simulink model "model"  (R2018b)
settings: Solver=VariableStepAuto  StartTime=0.0  StopTime=10.0  RelTol=1e-3
values from neighbouring files (symbols this model uses):
  dt = 0    [runScript.m]
  Vx = 0    [runScript.m]
  Vx_prev = 0    [runScript.m]
  Vy = 0    [runScript.m]
  Vy_prev = 0    [runScript.m]
  Vz = 0    [runScript.m]
  Vz_prev = 0    [runScript.m]
settings Model: Creator=Leshi  LastModifiedBy=Leshi

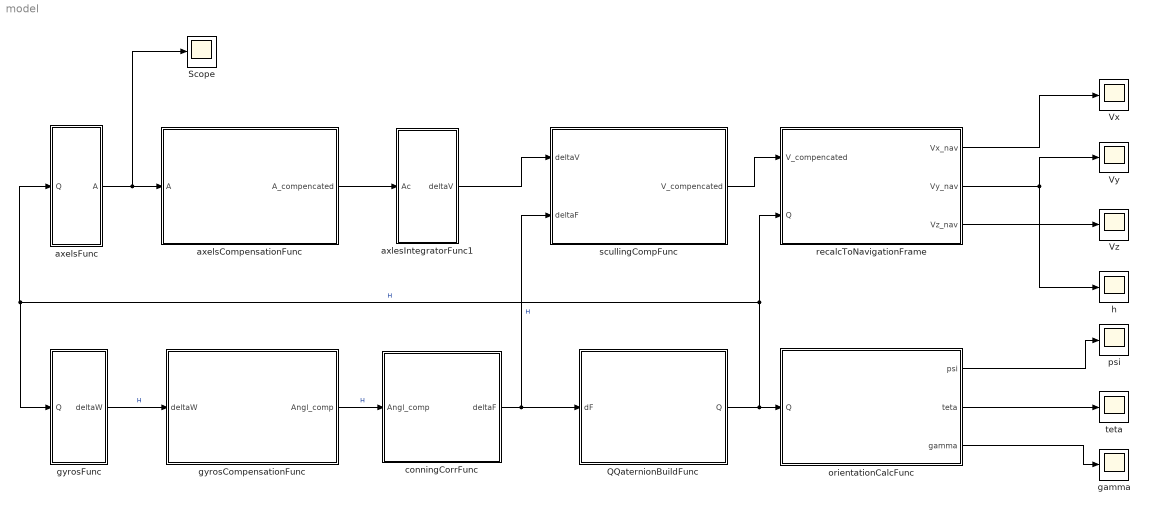
== system model ==
  QQaternionBuildFunc : MATLAB Function  TreatAsAtomicUnit=on
  Scope : Scope
  Vx : Scope
  Vy : Scope
  Vz : Scope
  axelsCompensationFunc : MATLAB Function  TreatAsAtomicUnit=on
  axelsFunc : MATLAB Function  TreatAsAtomicUnit=on
  axlesIntegratorFunc1 : MATLAB Function  TreatAsAtomicUnit=on
  conningCorrFunc : MATLAB Function  TreatAsAtomicUnit=on
  gamma : Scope
  gyrosCompensationFunc : MATLAB Function  TreatAsAtomicUnit=on
  gyrosFunc : MATLAB Function  TreatAsAtomicUnit=on
  h : Scope
  orientationCalcFunc : MATLAB Function  TreatAsAtomicUnit=on
  psi : Scope
  recalcToNavigationFrame : MATLAB Function  TreatAsAtomicUnit=on
  scullingCompFunc : MATLAB Function  TreatAsAtomicUnit=on
  teta : Scope
  wires:
  gyrosFunc/1(deltaW) -> gyrosCompensationFunc/1(deltaW)  "н"
  QQaternionBuildFunc/1(Q) -> orientationCalcFunc/1(Q), recalcToNavigationFrame/2(Q), gyrosFunc/1(Q), axelsFunc/1(Q)  "н"
  recalcToNavigationFrame/1(Vx_nav) -> Vx/1
  recalcToNavigationFrame/3(Vz_nav) -> Vz/1
  recalcToNavigationFrame/2(Vy_nav) -> h/1, Vy/1
  orientationCalcFunc/1(psi) -> psi/1
  orientationCalcFunc/2(teta) -> teta/1
  orientationCalcFunc/3(gamma) -> gamma/1
  gyrosCompensationFunc/1(Angl_comp) -> conningCorrFunc/1(Angl_comp)  "н"
  axlesIntegratorFunc1/1(deltaV) -> scullingCompFunc/1(deltaV)
  axelsFunc/1(A) -> Scope/1, axelsCompensationFunc/1(A)
  axelsCompensationFunc/1(A_compencated) -> axlesIntegratorFunc1/1(Ac)
  scullingCompFunc/1(V_compencated) -> recalcToNavigationFrame/1(V_compencated)
  conningCorrFunc/1(deltaF) -> scullingCompFunc/2(deltaF), QQaternionBuildFunc/1(dF)  "н"

== matlab function model/gyrosFunc ==
  data: deltaW output size=[1, 3]; Q input size=[1, 4]
% Give increment of anular vels
function deltaW = Gyros(Q)



Wx = awgn(0,10,'measured');
Wy = awgn(0,10,'measured');
Wz = awgn(0,10,'measured');

deltaW = [Wx, Wy, Wz];

== matlab function model/axelsFunc ==
  data: Q input size=[1, 4]; A output size=[1, 3]; g parameter
% Give pure aceleration
function A = Axels(Q, g)

[q0, q1, q2, q3] = parts(Q)
Q_ = quaternion(q0, -q1, -q2, -q3);
gCurrnet = Q * g * Q_;

Ax = awgn(gCurrnet(1),10,'measured');
Ay = awgn(gCurrnet(2),10,'measured');
Az = awgn(gCurrnet(3),10,'measured');

A = [Ax, Ay, Az];

== matlab function model/axelsCompensationFunc ==
  data: A input size=[1, 3]; A_compencated output; g parameter
function A_compencated  = AxelsCompensation(A, g)
Ax_compencated = A(1);
Ay_compencated = A(2) - g;
Az_compencated = A(3);

A_compencated = [Ax_compencated, Ay_compencated, Az_compencated];

== matlab function model/gyrosCompensationFunc ==
  data: Angl_comp output size=[1, 3]; deltaW input size=[1, 3]
% Returns compencated increment of angulag vel
function Angl_comp = GyrosCompensation(deltaW)
Wx_c = deltaW(1);
Wy_c = deltaW(2);
Wz_c = deltaW(3);

Angl_comp= [Wx_c, Wy_c, Wz_c];

== matlab function model/scullingCompFunc ==
  data: deltaV input size=[1, 3]; deltaF input; V_compencated output size=[1, 3]; Vx parameter; Vy parameter; Vz parameter; Vx_prev parameter; Vy_prev parameter; Vz_prev parameter
function V_compencated = ScullingCompensation(deltaV, deltaF, Vx, Vy, Vz, Vx_prev, Vy_prev, Vz_prev)
Vx = Vx_prev + Vy_prev * deltaF(3) - Vz_prev * deltaF(2) + deltaV(1);
Vy = Vy_prev + Vz_prev * deltaF(1) - Vx_prev * deltaF(3) + deltaV(2);
Vz = Vz_prev + Vx_prev * deltaF(2) - Vy_prev * deltaF(1) + deltaV(3);

Vx_prev = Vx;
Vy_prev = Vy;
Vz_prev = Vz;

V_compencated = [Vx, Vy, Vz];

== matlab function model/recalcToNavigationFrame ==
  data: V_compencated input size=[1, 3]; Vx_nav output; Q input size=[1, 4]; Vy_nav output; Vz_nav output
function [Vx_nav, Vy_nav, Vz_nav] = BodyToNavCalc(V_compencated, Q)

[q0, q1, q2, q3] = parts(Q);
Q_ = quaternion(q0, -q1, -q2, -q3);
V_nav = Q .* V_compencated .* Q_;

Vx_nav = V_nav(1);
Vy_nav = V_nav(2);
Vz_nav = V_nav(3);

== matlab function model/QQaternionBuildFunc ==
  data: Q output size=[1, 4]; dF input size=[1, 3]
function Q = QQaternionBuild(dF)

dL = quaternion();

Q = Q * dL;

% P = quaternion(cos(psi/2), 0, sin(psi/2), 0);
% Q = quaternion(cos(teta/2), 0, 0, sin(teta/2));
% R = quaternion(cos(gamma/2), sin(gamma/2), 0, 0);
% 
% C = P*Q*R;

== matlab function model/conningCorrFunc ==
  data: deltaF output size=[1, 3]; Angl_comp input size=[1, 3]
% Returns compencated increment of angulag vel
function deltaF  = ConingCorrection(Angl_comp)
dFx = Angl_comp(1);
dFy = Angl_comp(2);
dFz = Angl_comp(3);

deltaF = [dFx, dFy, dFz];

== matlab function model/orientationCalcFunc ==
  data: psi output; Q input size=[1,4]; teta output; gamma output
function [psi, teta, gamma] = OrientationAnglesCalc(Q)

% teta = atan2(C(3, 2), sqrt(C(3,1)^2 + C(3, 3)^2));
% psi = atan2(C(1,2), C(2,2));
% gamma = - atan2(C(3, 1), C(3, 3));

[q0, q1, q2, q3] = parts(Q);

psi = atan2(- (2 * q1 * q3  - 2 * q0 * q2), (2 * q1^2  + 2 * q0^2 - 1));
teta = asin(2 * q1 * q2  + 2 * q0 * q3);
gamma = atan2( - (2 * q2 * q3 - 2 * q0 * q1), (2 * q0^2 + 2 * q2^2 - 1));

== matlab function model/axlesIntegratorFunc1 ==
  data: Ac input size=[1, 3]; deltaV output size=[1, 3]; Vx parameter; Vz parameter; Vy parameter; dt parameter
function deltaV = AIntegrator(Ac, Vx, Vz, Vy, dt)
Vx = Ac(1) * dt;
Vy = Ac(2) * dt;
Vz = Ac(3) * dt;

deltaV = [Vx, Vy, Vz];
